simulink model "Aula3_Ex2Simulink"  (R2019b)
settings: Solver=VariableStepAuto  StartTime=0.0  StopTime=10.0  RelTol=1e-3
values from neighbouring files (symbols this model uses):
  D = DVect(2)    [aula3.m]    (also in aula3_mica.m = Dvector(n); s23.m = 0.1)
  K = 1    [aula3.m]
  M = 1    [aula3.m]    (also in aula3_mica.m)
settings Model: Creator=Emanuel Pereira  LastModifiedBy=Emanuel Pereira

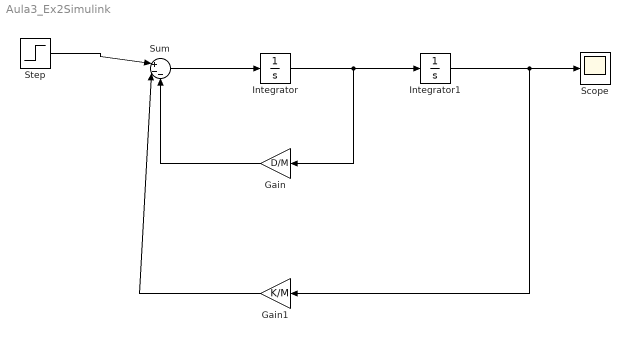
== system Aula3_Ex2Simulink ==
  Gain : Gain  Gain=D/M
  Gain1 : Gain  Gain=K/M
  Integrator : Integrator
  Integrator1 : Integrator
  Scope : Scope
  Step : Step  SampleTime=0
  Sum : Sum  Inputs=|+--
  wires:
  Sum/1 -> Integrator/1
  Integrator/1 -> Gain/1, Integrator1/1
  Integrator1/1 -> Gain1/1, Scope/1
  Gain1/1 -> Sum/2
  Gain/1 -> Sum/3
  Step/1 -> Sum/1
